simulink model "crazyflie_identic_articol"  (R2014b)
settings: Solver=ode45  StartTime=0.0  StopTime=150  RelTol=1e-4
undefined symbols (not defined in the file or in its folder): A, B, C, D
libraries: simulink x9
settings Model: Creator=uidd7441  LastModifiedBy=uidd7441
settings SolverCC: ZeroCrossAlgorithm=Adaptive  SolverResetMethod=Robust

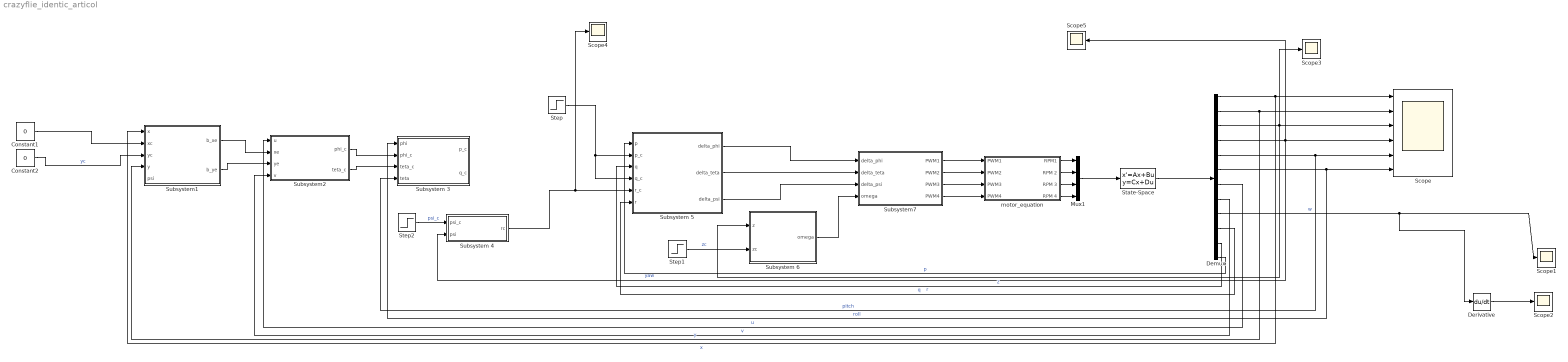
== system crazyflie_identic_articol ==
  Constant1 : Constant  Value=0
  Constant2 : Constant  Value=0
  Demux : Demux  Outputs=12
  Derivative : Derivative
  Mux1 : Mux
  Scope : Scope  NumInputPorts=6
      settings: YMin=0~0~0~0~0~-4e+06  YMax=2e+08~2e+08~1000~400000~4e+06~0
  Scope{1..5} (5 alike) : Scope
      Scope2 settings: SaveName=ScopeData2
      Scope3 settings: SaveName=ScopeData3
      Scope4 settings: YMin=-4e+06  YMax=-500000  SaveName=ScopeData4  MaxDataPoints=5000000
      Scope5 settings: TimeRange=2.494596015329648  YMin=250000  YMax=450000  SaveName=ScopeData5  MaxDataPoints=5000000
  State-Space : StateSpace  A=A  B=B  C=C  D=D  X0=[0 0 0 0 0 0 0 0 0 0 0 0]
  Step : Step  Time=0  After=0  SampleTime=0
  Step1 : Step  Time=0  After=0  SampleTime=0
  Step2 : Step  Time=0  After=0  SampleTime=0
  Subsystem 3 : Subsystem
  Subsystem 4 : Subsystem
  Subsystem 5 : Subsystem
  Subsystem 6 : Subsystem
  Subsystem1 : Subsystem
  Subsystem2 : Subsystem
  Subsystem7 : Subsystem
  motor_equation : Subsystem
  wires:
  Step1/1 -> Subsystem 6/2(zc)  "zc"
  Constant2/1 -> Subsystem1/3(yc)  "yc"
  Step2/1 -> Subsystem 4/1(psi_c)  "psi_c"
  Subsystem1/2(b_ye) -> Subsystem2/3(ye)
  Subsystem2/1(phi_c) -> Subsystem 3/2(phi_c)
  Subsystem2/2(teta_c) -> Subsystem 3/3(teta_c)
  Subsystem 4/1(rc) -> Scope4/1, Subsystem 5/5(r_c)
  Subsystem 6/1(omega) -> Subsystem7/4(omega)
  Subsystem7/1(PWM1) -> motor_equation/1(PWM1)
  Subsystem7/2(PWM2) -> motor_equation/2(PWM2)
  Subsystem7/3(PWM3) -> motor_equation/3(PWM3)
  Subsystem7/4(PWM4) -> motor_equation/4(PWM4)
  State-Space/1 -> Demux/1
  motor_equation/1("RPM1 ") -> Mux1/1
  motor_equation/2(RPM 2) -> Mux1/2
  motor_equation/3(RPM 3) -> Mux1/3
  motor_equation/4(RPM 4) -> Mux1/4
  Mux1/1 -> State-Space/1
  Subsystem1/1(b_xe) -> Subsystem2/2(xe)
  Constant1/1 -> Subsystem1/2(xc)
  Demux/3 -> Scope3/1, Subsystem 6/1(z), Scope/3  "z"
  Demux/1 -> Subsystem1/1(x), Scope/1  "x"
  Demux/2 -> Subsystem1/4(y), Scope/2  "y"
  Demux/4 -> Scope5/1, Subsystem 4/2(psi), Scope/4  "yaw"
  Demux/5 -> Subsystem 3/4(teta), Scope/5  "pitch"
  Demux/6 -> Subsystem 3/1("phi "), Scope/6  "roll"
  Demux/7 -> Subsystem2/1(u)  "u"
  Demux/8 -> Subsystem2/4(v)  "v"
  Demux/9 -> Derivative/1, Scope1/1  "w"
  Demux/11 -> Subsystem 5/3(q)  "q"
  Demux/12 -> Subsystem 5/1(p)  "p"
  Demux/10 -> Subsystem 5/6(r)  "r"
  Derivative/1 -> Scope2/1
  Subsystem 5/1(delta_phi) -> Subsystem7/1(delta_phi)
  Subsystem 5/2(delta_teta) -> Subsystem7/2(delta_teta)
  Subsystem 5/3(delta_psi) -> Subsystem7/3(delta_psi)
  Step/1 -> Subsystem 5/4(q_c), Subsystem 5/2(p_c)

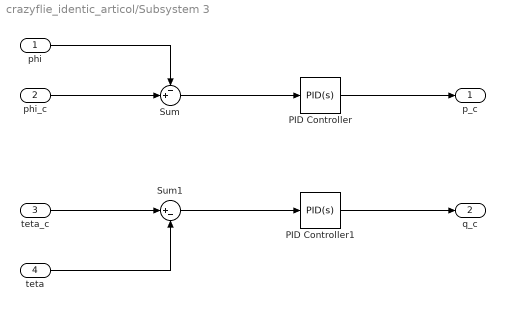
== system crazyflie_identic_articol/Subsystem 3 ==
  "phi " : Inport
  phi_c : Inport  Port=2
  teta_c : Inport  Port=3
  teta : Inport  Port=4
  PID Controller : simulink/Continuous/PID Controller  Controller=PID  TimeDomain=Continuous-time  SampleTime=-1  IntegratorMethod=Forward Euler  FilterMethod=Forward Euler  Form=Parallel  P=3.5  I=2  D=0  N=100  InitialConditionSource=internal  InitialConditionForIntegrator=0  InitialConditionForFilter=0  ExternalReset=none  LimitOutput=off  UpperSaturationLimit=inf  LowerSaturationLimit=-inf  LinearizeAsGain=on  AntiWindupMode=none  Kb=1  TrackingMode=off  Kt=1  PParamMin=[]  PParamMax=[]  IParamMin=[]  IParamMax=[]  DParamMin=[]  DParamMax=[]  NParamMin=[]  NParamMax=[]  KbParamMin=[]  KbParamMax=[]  KtParamMin=[]  KtParamMax=[]  POutMin=[]  POutMax=[]  IOutMin=[]  IOutMax=[]  DOutMin=[]  DOutMax=[]  NOutMin=[]  NOutMax=[]  KbOutMin=[]  KbOutMax=[]  KtOutMin=[]  KtOutMax=[]  IntegratorOutMin=[]  IntegratorOutMax=[]  FilterOutMin=[]  FilterOutMax=[]  SumOutMin=[]  SumOutMax=[]  SumI1OutMin=[]  SumI1OutMax=[]  SumI2OutMin=[]  SumI2OutMax=[]  SumI3OutMin=[]  SumI3OutMax=[]  SumDOutMin=[]  SumDOutMax=[]  SaturationOutMin=[]  SaturationOutMax=[]  IntegratorContinuousStateAttributes=''  IntegratorStateMustResolveToSignalObject=off  IntegratorRTWStateStorageClass=Auto  FilterContinuousStateAttributes=''  FilterStateMustResolveToSignalObject=off  FilterRTWStateStorageClass=Auto  DifferentiatorICPrevScaledInput=0  DifferentiatorOutMin=[]  DifferentiatorOutMax=[]  UseFilter=on
  PID Controller1 : simulink/Continuous/PID Controller  Controller=PID  TimeDomain=Continuous-time  SampleTime=-1  IntegratorMethod=Forward Euler  FilterMethod=Forward Euler  Form=Parallel  P=3.5  I=2  D=0  N=100  InitialConditionSource=internal  InitialConditionForIntegrator=0  InitialConditionForFilter=0  ExternalReset=none  LimitOutput=off  UpperSaturationLimit=inf  LowerSaturationLimit=-inf  LinearizeAsGain=on  AntiWindupMode=none  Kb=1  TrackingMode=off  Kt=1  PParamMin=[]  PParamMax=[]  IParamMin=[]  IParamMax=[]  DParamMin=[]  DParamMax=[]  NParamMin=[]  NParamMax=[]  KbParamMin=[]  KbParamMax=[]  KtParamMin=[]  KtParamMax=[]  POutMin=[]  POutMax=[]  IOutMin=[]  IOutMax=[]  DOutMin=[]  DOutMax=[]  NOutMin=[]  NOutMax=[]  KbOutMin=[]  KbOutMax=[]  KtOutMin=[]  KtOutMax=[]  IntegratorOutMin=[]  IntegratorOutMax=[]  FilterOutMin=[]  FilterOutMax=[]  SumOutMin=[]  SumOutMax=[]  SumI1OutMin=[]  SumI1OutMax=[]  SumI2OutMin=[]  SumI2OutMax=[]  SumI3OutMin=[]  SumI3OutMax=[]  SumDOutMin=[]  SumDOutMax=[]  SaturationOutMin=[]  SaturationOutMax=[]  IntegratorContinuousStateAttributes=''  IntegratorStateMustResolveToSignalObject=off  IntegratorRTWStateStorageClass=Auto  FilterContinuousStateAttributes=''  FilterStateMustResolveToSignalObject=off  FilterRTWStateStorageClass=Auto  DifferentiatorICPrevScaledInput=0  DifferentiatorOutMin=[]  DifferentiatorOutMax=[]  UseFilter=on
  Sum : Sum  Inputs=-+|
  Sum1 : Sum  Inputs=|+-
  p_c : Outport
  q_c : Outport  Port=2
  wires:
  "phi "/1 -> Sum/1
  phi_c/1 -> Sum/2
  teta_c/1 -> Sum1/1
  teta/1 -> Sum1/2
  Sum/1 -> PID Controller/1
  Sum1/1 -> PID Controller1/1
  PID Controller/1 -> p_c/1
  PID Controller1/1 -> q_c/1

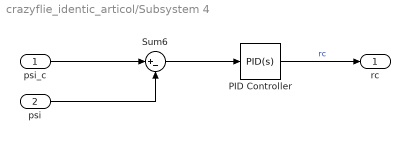
== system crazyflie_identic_articol/Subsystem 4 ==
  psi_c : Inport
  psi : Inport  Port=2
  PID Controller : simulink/Continuous/PID Controller  Controller=PID  TimeDomain=Continuous-time  SampleTime=-1  IntegratorMethod=Forward Euler  FilterMethod=Forward Euler  Form=Parallel  P=3  I=0  D=0  N=0  InitialConditionSource=internal  InitialConditionForIntegrator=0  InitialConditionForFilter=0  ExternalReset=none  LimitOutput=off  UpperSaturationLimit=inf  LowerSaturationLimit=-inf  LinearizeAsGain=on  AntiWindupMode=none  Kb=1  TrackingMode=off  Kt=1  PParamMin=[]  PParamMax=[]  IParamMin=[]  IParamMax=[]  DParamMin=[]  DParamMax=[]  NParamMin=[]  NParamMax=[]  KbParamMin=[]  KbParamMax=[]  KtParamMin=[]  KtParamMax=[]  POutMin=[]  POutMax=[]  IOutMin=[]  IOutMax=[]  DOutMin=[]  DOutMax=[]  NOutMin=[]  NOutMax=[]  KbOutMin=[]  KbOutMax=[]  KtOutMin=[]  KtOutMax=[]  IntegratorOutMin=[]  IntegratorOutMax=[]  FilterOutMin=[]  FilterOutMax=[]  SumOutMin=[]  SumOutMax=[]  SumI1OutMin=[]  SumI1OutMax=[]  SumI2OutMin=[]  SumI2OutMax=[]  SumI3OutMin=[]  SumI3OutMax=[]  SumDOutMin=[]  SumDOutMax=[]  SaturationOutMin=[]  SaturationOutMax=[]  IntegratorContinuousStateAttributes=''  IntegratorStateMustResolveToSignalObject=off  IntegratorRTWStateStorageClass=Auto  FilterContinuousStateAttributes=''  FilterStateMustResolveToSignalObject=off  FilterRTWStateStorageClass=Auto  DifferentiatorICPrevScaledInput=0  DifferentiatorOutMin=[]  DifferentiatorOutMax=[]  UseFilter=on
  Sum6 : Sum  Inputs=|+-
  rc : Outport
  wires:
  Sum6/1 -> PID Controller/1
  PID Controller/1 -> rc/1  "rc"
  psi_c/1 -> Sum6/1
  psi/1 -> Sum6/2

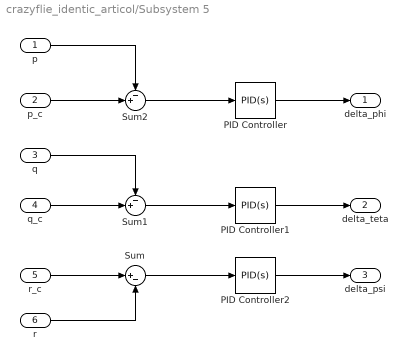
== system crazyflie_identic_articol/Subsystem 5 ==
  p : Inport
  p_c : Inport  Port=2
  q : Inport  Port=3
  q_c : Inport  Port=4
  r_c : Inport  Port=5
  r : Inport  Port=6
  PID Controller : simulink/Continuous/PID Controller  Controller=PID  TimeDomain=Continuous-time  SampleTime=-1  IntegratorMethod=Forward Euler  FilterMethod=Forward Euler  Form=Parallel  P=70  I=0  D=0  N=100  InitialConditionSource=internal  InitialConditionForIntegrator=0  InitialConditionForFilter=0  ExternalReset=none  LimitOutput=off  UpperSaturationLimit=inf  LowerSaturationLimit=-inf  LinearizeAsGain=on  AntiWindupMode=none  Kb=1  TrackingMode=off  Kt=1  PParamMin=[]  PParamMax=[]  IParamMin=[]  IParamMax=[]  DParamMin=[]  DParamMax=[]  NParamMin=[]  NParamMax=[]  KbParamMin=[]  KbParamMax=[]  KtParamMin=[]  KtParamMax=[]  POutMin=[]  POutMax=[]  IOutMin=[]  IOutMax=[]  DOutMin=[]  DOutMax=[]  NOutMin=[]  NOutMax=[]  KbOutMin=[]  KbOutMax=[]  KtOutMin=[]  KtOutMax=[]  IntegratorOutMin=[]  IntegratorOutMax=[]  FilterOutMin=[]  FilterOutMax=[]  SumOutMin=[]  SumOutMax=[]  SumI1OutMin=[]  SumI1OutMax=[]  SumI2OutMin=[]  SumI2OutMax=[]  SumI3OutMin=[]  SumI3OutMax=[]  SumDOutMin=[]  SumDOutMax=[]  SaturationOutMin=[]  SaturationOutMax=[]  IntegratorContinuousStateAttributes=''  IntegratorStateMustResolveToSignalObject=off  IntegratorRTWStateStorageClass=Auto  FilterContinuousStateAttributes=''  FilterStateMustResolveToSignalObject=off  FilterRTWStateStorageClass=Auto  DifferentiatorICPrevScaledInput=0  DifferentiatorOutMin=[]  DifferentiatorOutMax=[]  UseFilter=on
  PID Controller1 : simulink/Continuous/PID Controller  Controller=PID  TimeDomain=Continuous-time  SampleTime=-1  IntegratorMethod=Forward Euler  FilterMethod=Forward Euler  Form=Parallel  P=70  I=0  D=0  N=100  InitialConditionSource=internal  InitialConditionForIntegrator=0  InitialConditionForFilter=0  ExternalReset=none  LimitOutput=off  UpperSaturationLimit=inf  LowerSaturationLimit=-inf  LinearizeAsGain=on  AntiWindupMode=none  Kb=1  TrackingMode=off  Kt=1  PParamMin=[]  PParamMax=[]  IParamMin=[]  IParamMax=[]  DParamMin=[]  DParamMax=[]  NParamMin=[]  NParamMax=[]  KbParamMin=[]  KbParamMax=[]  KtParamMin=[]  KtParamMax=[]  POutMin=[]  POutMax=[]  IOutMin=[]  IOutMax=[]  DOutMin=[]  DOutMax=[]  NOutMin=[]  NOutMax=[]  KbOutMin=[]  KbOutMax=[]  KtOutMin=[]  KtOutMax=[]  IntegratorOutMin=[]  IntegratorOutMax=[]  FilterOutMin=[]  FilterOutMax=[]  SumOutMin=[]  SumOutMax=[]  SumI1OutMin=[]  SumI1OutMax=[]  SumI2OutMin=[]  SumI2OutMax=[]  SumI3OutMin=[]  SumI3OutMax=[]  SumDOutMin=[]  SumDOutMax=[]  SaturationOutMin=[]  SaturationOutMax=[]  IntegratorContinuousStateAttributes=''  IntegratorStateMustResolveToSignalObject=off  IntegratorRTWStateStorageClass=Auto  FilterContinuousStateAttributes=''  FilterStateMustResolveToSignalObject=off  FilterRTWStateStorageClass=Auto  DifferentiatorICPrevScaledInput=0  DifferentiatorOutMin=[]  DifferentiatorOutMax=[]  UseFilter=on
  PID Controller2 : simulink/Continuous/PID Controller  Controller=PID  TimeDomain=Continuous-time  SampleTime=-1  IntegratorMethod=Forward Euler  FilterMethod=Forward Euler  Form=Parallel  P=70  I=16.7  D=0  N=100  InitialConditionSource=internal  InitialConditionForIntegrator=0  InitialConditionForFilter=0  ExternalReset=none  LimitOutput=off  UpperSaturationLimit=inf  LowerSaturationLimit=-inf  LinearizeAsGain=on  AntiWindupMode=none  Kb=1  TrackingMode=off  Kt=1  PParamMin=[]  PParamMax=[]  IParamMin=[]  IParamMax=[]  DParamMin=[]  DParamMax=[]  NParamMin=[]  NParamMax=[]  KbParamMin=[]  KbParamMax=[]  KtParamMin=[]  KtParamMax=[]  POutMin=[]  POutMax=[]  IOutMin=[]  IOutMax=[]  DOutMin=[]  DOutMax=[]  NOutMin=[]  NOutMax=[]  KbOutMin=[]  KbOutMax=[]  KtOutMin=[]  KtOutMax=[]  IntegratorOutMin=[]  IntegratorOutMax=[]  FilterOutMin=[]  FilterOutMax=[]  SumOutMin=[]  SumOutMax=[]  SumI1OutMin=[]  SumI1OutMax=[]  SumI2OutMin=[]  SumI2OutMax=[]  SumI3OutMin=[]  SumI3OutMax=[]  SumDOutMin=[]  SumDOutMax=[]  SaturationOutMin=[]  SaturationOutMax=[]  IntegratorContinuousStateAttributes=''  IntegratorStateMustResolveToSignalObject=off  IntegratorRTWStateStorageClass=Auto  FilterContinuousStateAttributes=''  FilterStateMustResolveToSignalObject=off  FilterRTWStateStorageClass=Auto  DifferentiatorICPrevScaledInput=0  DifferentiatorOutMin=[]  DifferentiatorOutMax=[]  UseFilter=on
  Sum : Sum  Inputs=|+-
  Sum1 : Sum  Inputs=-+|
  Sum2 : Sum  Inputs=-+|
  delta_phi : Outport
  delta_teta : Outport  Port=2
  delta_psi : Outport  Port=3
  wires:
  q/1 -> Sum1/1
  q_c/1 -> Sum1/2
  p_c/1 -> Sum2/2
  p/1 -> Sum2/1
  r_c/1 -> Sum/1
  r/1 -> Sum/2
  Sum2/1 -> PID Controller/1
  Sum1/1 -> PID Controller1/1
  Sum/1 -> PID Controller2/1
  PID Controller/1 -> delta_phi/1
  PID Controller1/1 -> delta_teta/1
  PID Controller2/1 -> delta_psi/1

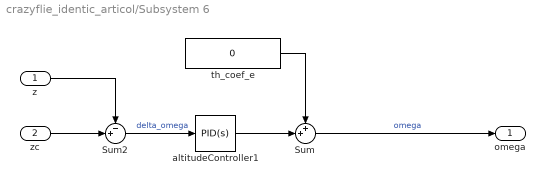
== system crazyflie_identic_articol/Subsystem 6 ==
  z : Inport
  zc : Inport  Port=2
  Sum : Sum  Inputs=++|
  Sum2 : Sum  Inputs=-+|
  altitudeController1 : simulink/Continuous/PID Controller  Controller=PID  TimeDomain=Continuous-time  SampleTime=-1  IntegratorMethod=Forward Euler  FilterMethod=Forward Euler  Form=Parallel  P=11000  I=3500  D=9000  N=100  InitialConditionSource=internal  InitialConditionForIntegrator=0  InitialConditionForFilter=0  ExternalReset=none  LimitOutput=off  UpperSaturationLimit=20000  LowerSaturationLimit=-15000  LinearizeAsGain=on  AntiWindupMode=none  Kb=1  TrackingMode=off  Kt=1  PParamMin=[]  PParamMax=[]  IParamMin=[]  IParamMax=[]  DParamMin=[]  DParamMax=[]  NParamMin=[]  NParamMax=[]  KbParamMin=[]  KbParamMax=[]  KtParamMin=[]  KtParamMax=[]  POutMin=[]  POutMax=[]  IOutMin=[]  IOutMax=[]  DOutMin=[]  DOutMax=[]  NOutMin=[]  NOutMax=[]  KbOutMin=[]  KbOutMax=[]  KtOutMin=[]  KtOutMax=[]  IntegratorOutMin=[]  IntegratorOutMax=[]  FilterOutMin=[]  FilterOutMax=[]  SumOutMin=[]  SumOutMax=[]  SumI1OutMin=[]  SumI1OutMax=[]  SumI2OutMin=[]  SumI2OutMax=[]  SumI3OutMin=[]  SumI3OutMax=[]  SumDOutMin=[]  SumDOutMax=[]  SaturationOutMin=[]  SaturationOutMax=[]  IntegratorContinuousStateAttributes=''  IntegratorStateMustResolveToSignalObject=off  IntegratorRTWStateStorageClass=Auto  FilterContinuousStateAttributes=''  FilterStateMustResolveToSignalObject=off  FilterRTWStateStorageClass=Auto  DifferentiatorICPrevScaledInput=0  DifferentiatorOutMin=[]  DifferentiatorOutMax=[]  UseFilter=on
  "th_coef_e " : Constant  Value=0
  omega : Outport
  wires:
  "th_coef_e "/1 -> Sum/1
  Sum/1 -> omega/1  "omega"
  zc/1 -> Sum2/2
  z/1 -> Sum2/1
  Sum2/1 -> altitudeController1/1  "delta_omega"
  altitudeController1/1 -> Sum/2

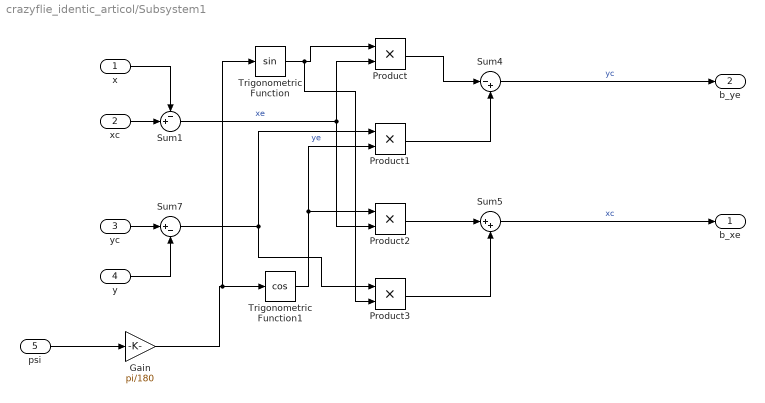
== system crazyflie_identic_articol/Subsystem1 ==
  x : Inport
  xc : Inport  Port=2
  yc : Inport  Port=3
  y : Inport  Port=4
  psi : Inport  Port=5
  Gain : Gain  Gain=pi/180
  Product{,1..3} (4 alike) : Product
  Sum1 : Sum  Inputs=-+|
  Sum4 : Sum  Inputs=|-+
  Sum5 : Sum  Inputs=|++
  Sum7 : Sum  Inputs=|+-
  Trigonometric Function : Trigonometry
  Trigonometric Function1 : Trigonometry  Operator=cos
  b_xe : Outport
  b_ye : Outport  Port=2
  wires:
  Sum1/1 -> Product/2, Product2/2  "xe"
  Sum7/1 -> Product1/1, Product3/1  "ye"
  Trigonometric Function/1 -> Product3/2, Product/1
  Product/1 -> Sum4/1
  Product1/1 -> Sum4/2
  Trigonometric Function1/1 -> Product1/2, Product2/1
  Product2/1 -> Sum5/1
  Product3/1 -> Sum5/2
  Sum4/1 -> b_ye/1  "yc"
  Sum5/1 -> b_xe/1  "xc"
  x/1 -> Sum1/1
  xc/1 -> Sum1/2
  yc/1 -> Sum7/1
  y/1 -> Sum7/2
  psi/1 -> Gain/1
  Gain/1 -> Trigonometric Function/1, Trigonometric Function1/1

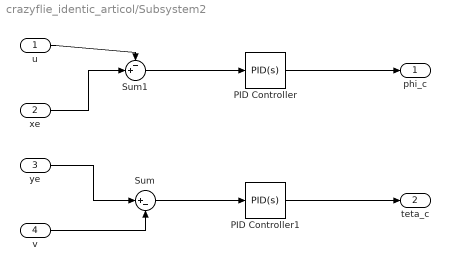
== system crazyflie_identic_articol/Subsystem2 ==
  u : Inport
  xe : Inport  Port=2
  ye : Inport  Port=3
  v : Inport  Port=4
  PID Controller : simulink/Continuous/PID Controller  Controller=PID  TimeDomain=Continuous-time  SampleTime=-1  IntegratorMethod=Forward Euler  FilterMethod=Forward Euler  Form=Parallel  P=30  I=2  D=0  N=0  InitialConditionSource=internal  InitialConditionForIntegrator=0  InitialConditionForFilter=0  ExternalReset=none  LimitOutput=on  UpperSaturationLimit=30  LowerSaturationLimit=-30  LinearizeAsGain=on  AntiWindupMode=none  Kb=1  TrackingMode=off  Kt=1  PParamMin=[]  PParamMax=[]  IParamMin=[]  IParamMax=[]  DParamMin=[]  DParamMax=[]  NParamMin=[]  NParamMax=[]  KbParamMin=[]  KbParamMax=[]  KtParamMin=[]  KtParamMax=[]  POutMin=[]  POutMax=[]  IOutMin=[]  IOutMax=[]  DOutMin=[]  DOutMax=[]  NOutMin=[]  NOutMax=[]  KbOutMin=[]  KbOutMax=[]  KtOutMin=[]  KtOutMax=[]  IntegratorOutMin=[]  IntegratorOutMax=[]  FilterOutMin=[]  FilterOutMax=[]  SumOutMin=[]  SumOutMax=[]  SumI1OutMin=[]  SumI1OutMax=[]  SumI2OutMin=[]  SumI2OutMax=[]  SumI3OutMin=[]  SumI3OutMax=[]  SumDOutMin=[]  SumDOutMax=[]  SaturationOutMin=[]  SaturationOutMax=[]  IntegratorContinuousStateAttributes=''  IntegratorStateMustResolveToSignalObject=off  IntegratorRTWStateStorageClass=Auto  FilterContinuousStateAttributes=''  FilterStateMustResolveToSignalObject=off  FilterRTWStateStorageClass=Auto  DifferentiatorICPrevScaledInput=0  DifferentiatorOutMin=[]  DifferentiatorOutMax=[]  UseFilter=on
  PID Controller1 : simulink/Continuous/PID Controller  Controller=PID  TimeDomain=Continuous-time  SampleTime=-1  IntegratorMethod=Forward Euler  FilterMethod=Forward Euler  Form=Parallel  P=-30  I=-2  D=0  N=100  InitialConditionSource=internal  InitialConditionForIntegrator=0  InitialConditionForFilter=0  ExternalReset=none  LimitOutput=on  UpperSaturationLimit=30  LowerSaturationLimit=-30  LinearizeAsGain=on  AntiWindupMode=none  Kb=1  TrackingMode=off  Kt=1  PParamMin=[]  PParamMax=[]  IParamMin=[]  IParamMax=[]  DParamMin=[]  DParamMax=[]  NParamMin=[]  NParamMax=[]  KbParamMin=[]  KbParamMax=[]  KtParamMin=[]  KtParamMax=[]  POutMin=[]  POutMax=[]  IOutMin=[]  IOutMax=[]  DOutMin=[]  DOutMax=[]  NOutMin=[]  NOutMax=[]  KbOutMin=[]  KbOutMax=[]  KtOutMin=[]  KtOutMax=[]  IntegratorOutMin=[]  IntegratorOutMax=[]  FilterOutMin=[]  FilterOutMax=[]  SumOutMin=[]  SumOutMax=[]  SumI1OutMin=[]  SumI1OutMax=[]  SumI2OutMin=[]  SumI2OutMax=[]  SumI3OutMin=[]  SumI3OutMax=[]  SumDOutMin=[]  SumDOutMax=[]  SaturationOutMin=[]  SaturationOutMax=[]  IntegratorContinuousStateAttributes=''  IntegratorStateMustResolveToSignalObject=off  IntegratorRTWStateStorageClass=Auto  FilterContinuousStateAttributes=''  FilterStateMustResolveToSignalObject=off  FilterRTWStateStorageClass=Auto  DifferentiatorICPrevScaledInput=0  DifferentiatorOutMin=[]  DifferentiatorOutMax=[]  UseFilter=on
  Sum : Sum  Inputs=|+-
  Sum1 : Sum  Inputs=-+|
  phi_c : Outport
  teta_c : Outport  Port=2
  wires:
  u/1 -> Sum1/1
  xe/1 -> Sum1/2
  ye/1 -> Sum/1
  v/1 -> Sum/2
  Sum/1 -> PID Controller1/1
  Sum1/1 -> PID Controller/1
  PID Controller/1 -> phi_c/1
  PID Controller1/1 -> teta_c/1

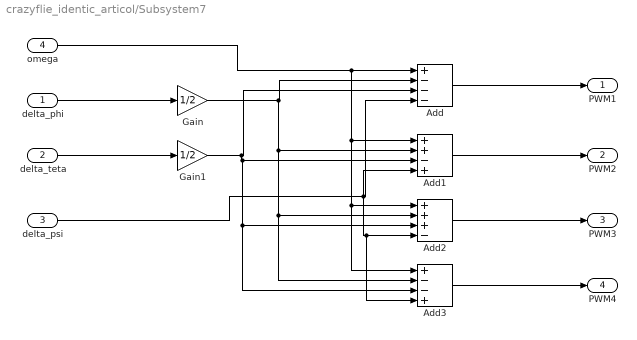
== system crazyflie_identic_articol/Subsystem7 ==
  delta_phi : Inport
  delta_teta : Inport  Port=2
  delta_psi : Inport  Port=3
  omega : Inport  Port=4
  Add : Sum  Inputs=+---
  Add1 : Sum  Inputs=++-+
  Add2 : Sum  Inputs=+++-
  Add3 : Sum  Inputs=+--+
  Gain : Gain  Gain=1/2
  Gain1 : Gain  Gain=1/2
  PWM1 : Outport
  PWM2 : Outport  Port=2
  PWM3 : Outport  Port=3
  PWM4 : Outport  Port=4
  wires:
  delta_phi/1 -> Gain/1
  delta_teta/1 -> Gain1/1
  Add/1 -> PWM1/1
  Add1/1 -> PWM2/1
  Add2/1 -> PWM3/1
  Add3/1 -> PWM4/1
  omega/1 -> Add3/1, Add2/1, Add1/1, Add/1
  Gain/1 -> Add3/2, Add2/2, Add1/2, Add/2
  Gain1/1 -> Add3/3, Add2/3, Add1/3, Add/3
  delta_psi/1 -> Add3/4, Add2/4, Add1/4, Add/4

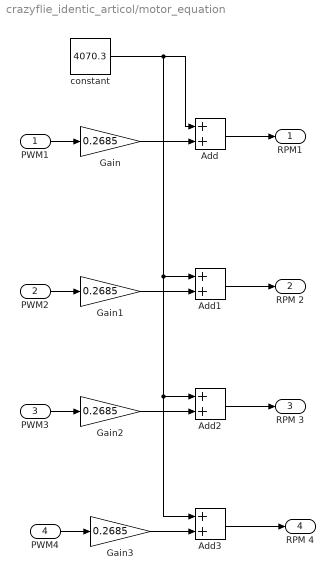
== system crazyflie_identic_articol/motor_equation ==
  PWM1 : Inport
  PWM2 : Inport  Port=2
  PWM3 : Inport  Port=3
  PWM4 : Inport  Port=4
  Add{,1..3} (4 alike) : Sum
  Gain{,1..3} (4 alike) : Gain  Gain=0.2685
  constant : Constant  Value=4070.3
  "RPM1 " : Outport
  RPM 2 : Outport  Port=2
  RPM 3 : Outport  Port=3
  RPM 4 : Outport  Port=4
  wires:
  constant/1 -> Add3/1, Add2/1, Add1/1, Add/1
  Gain/1 -> Add/2
  PWM1/1 -> Gain/1
  Add/1 -> "RPM1 "/1
  Gain1/1 -> Add1/2
  PWM2/1 -> Gain1/1
  Add1/1 -> RPM 2/1
  Gain2/1 -> Add2/2
  PWM3/1 -> Gain2/1
  Add2/1 -> RPM 3/1
  Gain3/1 -> Add3/2
  PWM4/1 -> Gain3/1
  Add3/1 -> RPM 4/1
